simulink model "CenterOfPressure_TestModel"  (R2014a)
settings: Solver=ode45  StartTime=0.0  StopTime=10.0  RelTol=1e-3
InitFcn:
  | fin_center_distance=1.7;
  | fin_root_chord=1.6;
  | fin_tip_chord=0.85;
  | d_nose_tip_to_fins=11.2;
  | fins_count=4;
  | height_fins=1.65;
  | diameter_outer=0.75;
  | height_nose_cone=3.6;
  | fin_sweep_length=0.75;
libraries: rocket_angular_flight_library x5
settings Model: Creator=scorpii  LastModifiedBy=scorpii

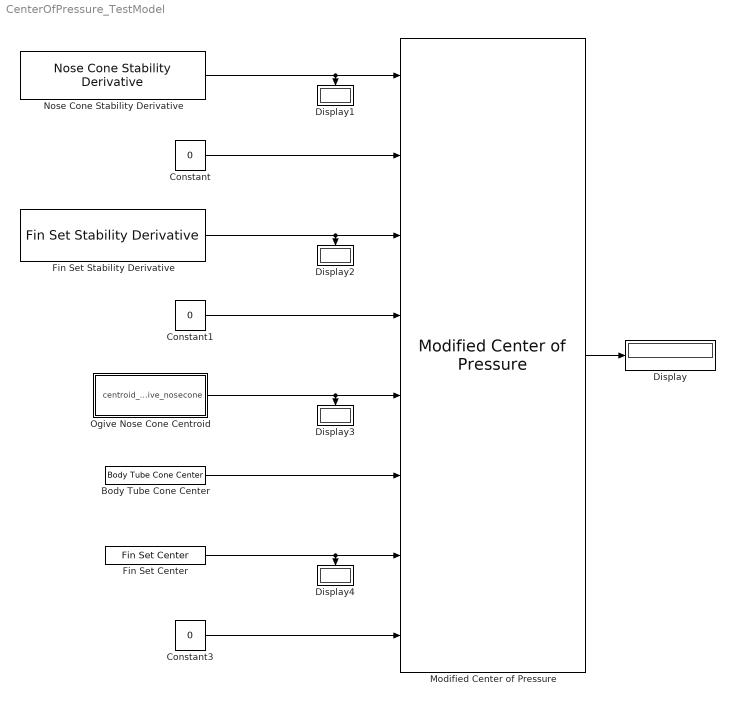
== system CenterOfPressure_TestModel ==
  Body Tube Cone Center : rocket_angular_flight_library/Center of Pressure/Body Tube Cone Center
  Constant : Constant  Value=0
  Constant1 : Constant  Value=0
  Constant3 : Constant  Value=0
  Display{,1..4} (5 alike) : Display
  Fin Set Center : rocket_angular_flight_library/Center of Pressure/Fin Set Center
  Fin Set Stability Derivative : rocket_angular_flight_library/Rocket Stability Derivative/Fin Set Stability Derivative
  Modified Center of Pressure : rocket_angular_flight_library/Center of Pressure/Modified Center of Pressure
  Nose Cone Stability Derivative : rocket_angular_flight_library/Rocket Stability Derivative/Nose Cone Stability Derivative
  Ogive Nose Cone Centroid : Subsystem
  wires:
  Modified Center of Pressure/1 -> Display/1
  Fin Set Stability Derivative/1 -> Display2/1, Modified Center of Pressure/3
  Constant/1 -> Modified Center of Pressure/2
  Constant1/1 -> Modified Center of Pressure/4
  Ogive Nose Cone Centroid/1(centroid_ogive_nosecone) -> Display3/1, Modified Center of Pressure/5
  Fin Set Center/1 -> Display4/1, Modified Center of Pressure/7
  Body Tube Cone Center/1 -> Modified Center of Pressure/6
  Constant3/1 -> Modified Center of Pressure/8
  Nose Cone Stability Derivative/1 -> Display1/1, Modified Center of Pressure/1

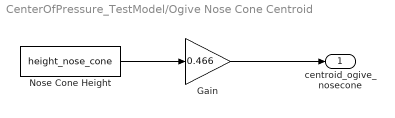
== system CenterOfPressure_TestModel/Ogive Nose Cone Centroid ==
  Gain : Gain  Gain=0.466
  Nose Cone Height : Constant  Value=height_nose_cone
  centroid_ogive_nosecone : Outport
  wires:
  Gain/1 -> centroid_ogive_nosecone/1
  Nose Cone Height/1 -> Gain/1
